simulink model "sim_stateEstimator"  (R2023b)
settings: Solver=VariableStepAuto  StartTime=0.0  StopTime=TSim  RelTol=1e-3
undefined symbols (not defined in the file): A, B, C, dampingCoeff, freqDist, initPos, initVel, K, l, magDist, mass, phaseDist, springCoeff
libraries: simulink x2
settings Model: Creator=uos  LastModifiedBy=hblee

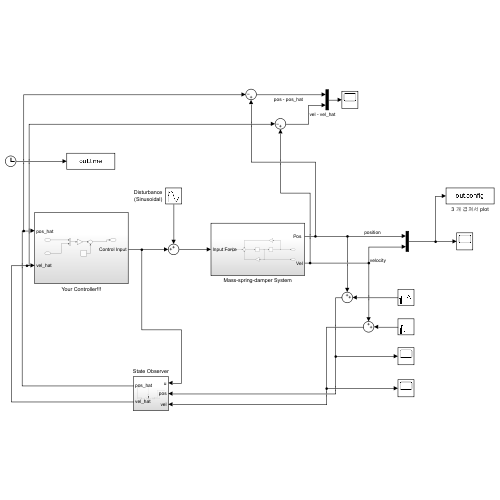
[thumbnail: Simulink's stored preview of the top-level diagram]
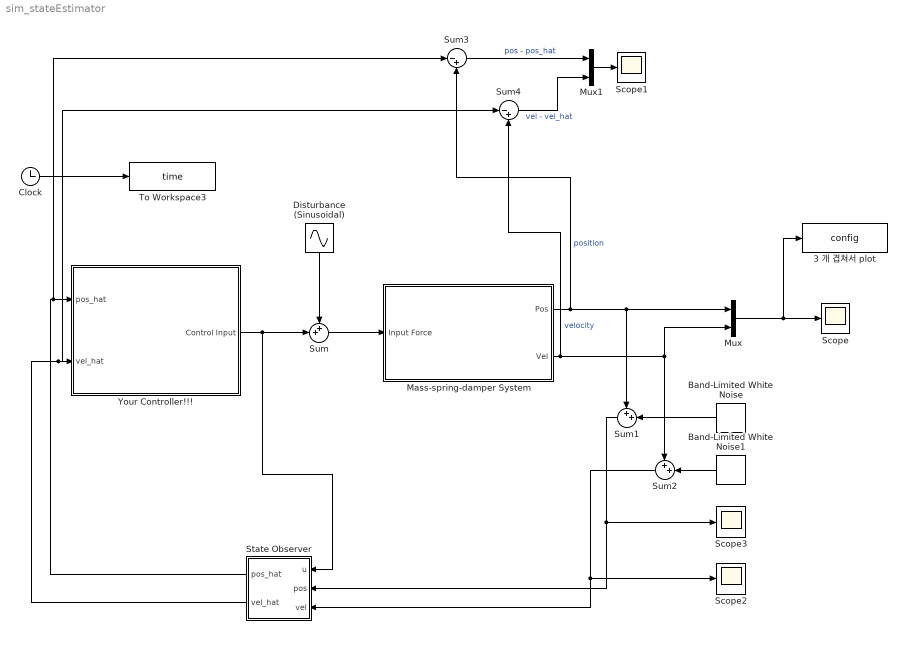
== system sim_stateEstimator ==
  3 개 겹쳐서 plot : ToWorkspace  VariableName=config  SampleTime=-1
  Band-Limited White Noise : simulink/Sources/Band-Limited White Noise  Cov=powerNoise  Ts=0.001  seed=[23341]
  Band-Limited White Noise1 : simulink/Sources/Band-Limited White Noise  Cov=powerNoise  Ts=0.001  seed=[23341]
  Clock : Clock
  Disturbance (Sinusoidal) : Sin  Amplitude=magDist  Bias=phaseDist  Frequency=freqDist  SampleTime=0
  Mass-spring-damper System : Subsystem
  Mux : Mux  Inputs=2
  Mux1 : Mux  Inputs=2
  Scope{,1..3} (4 alike) : Scope
  State Observer : Subsystem
  Sum : Sum  Inputs=++|
  Sum1 : Sum  Inputs=++|
  Sum2 : Sum  Inputs=++|
  Sum3 : Sum  Inputs=|-+
  Sum4 : Sum  Inputs=|-+
  To Workspace3 : ToWorkspace  VariableName=time  SampleTime=-1
  Your Controller!!! : Subsystem
  wires:
  Mass-spring-damper System/2(Vel) -> Mux/2, Sum2/1, Sum4/2  "velocity"
  Sum/1 -> Mass-spring-damper System/1("Input Force ")
  Your Controller!!!/1(Control Input) -> Sum/2, State Observer/1(u)
  Sum1/1 -> State Observer/2(pos), Scope3/1
  Sum2/1 -> State Observer/3(vel), Scope2/1
  Band-Limited White Noise/1 -> Sum1/2
  Band-Limited White Noise1/1 -> Sum2/2
  Disturbance (Sinusoidal)/1 -> Sum/1
  Clock/1 -> To Workspace3/1
  Mass-spring-damper System/1("Pos ") -> Sum3/2, Sum1/1, Mux/1  "position"
  Mux/1 -> 3 개 겹쳐서 plot/1, Scope/1
  State Observer/1(pos_hat) -> Sum3/1, Your Controller!!!/1(pos_hat)
  State Observer/2(vel_hat) -> Sum4/1, Your Controller!!!/2(vel_hat)
  Mux1/1 -> Scope1/1
  Sum3/1 -> Mux1/1  "pos - pos_hat"
  Sum4/1 -> Mux1/2  "vel - vel_hat"

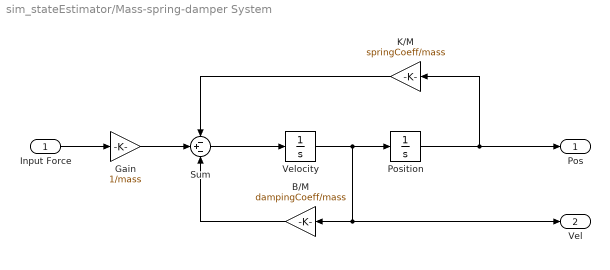
== system sim_stateEstimator/Mass-spring-damper System ==
  "Input Force " : Inport
  B/M : Gain  Gain=dampingCoeff/mass
  Gain : Gain  Gain=1/mass
  K/M : Gain  Gain=springCoeff/mass
  Position : Integrator  InitialCondition=initPos
  Sum : Sum  Inputs=-+-
  Velocity : Integrator  InitialCondition=initVel
  "Pos " : Outport
  Vel : Outport  Port=2
  wires:
  Velocity/1 -> Vel/1, B/M/1, Position/1
  Gain/1 -> Sum/2
  "Input Force "/1 -> Gain/1
  Position/1 -> "Pos "/1, K/M/1
  K/M/1 -> Sum/1
  B/M/1 -> Sum/3
  Sum/1 -> Velocity/1

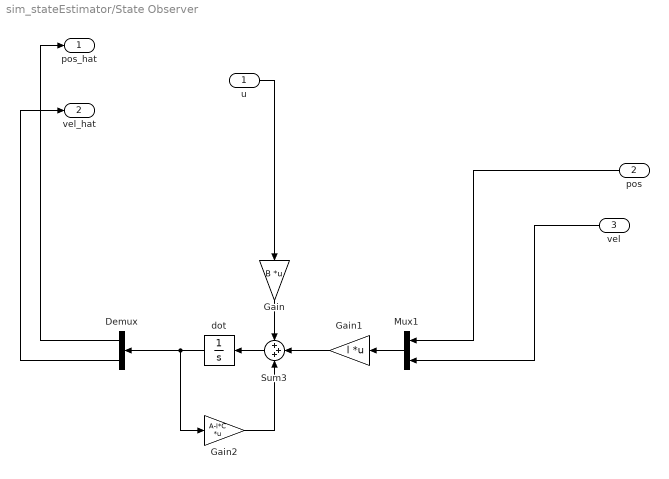
== system sim_stateEstimator/State Observer ==
  u : Inport
  pos : Inport  Port=2
  vel : Inport  Port=3
  Demux : Demux  Outputs=2
  Gain : Gain  Gain=B  Multiplication=Matrix(K*u)
  Gain1 : Gain  Gain=l  Multiplication=Matrix(K*u)
  Gain2 : Gain  Gain=A-l*C  Multiplication=Matrix(K*u)
  Mux1 : Mux  Inputs=2
  Sum3 : Sum  Inputs=+++
  dot : Integrator
  pos_hat : Outport
  vel_hat : Outport  Port=2
  wires:
  dot/1 -> Demux/1, Gain2/1
  pos/1 -> Mux1/1
  Mux1/1 -> Gain1/1
  Sum3/1 -> dot/1
  Gain2/1 -> Sum3/3
  Gain1/1 -> Sum3/2
  Gain/1 -> Sum3/1
  vel/1 -> Mux1/2
  Demux/2 -> vel_hat/1
  Demux/1 -> pos_hat/1
  u/1 -> Gain/1

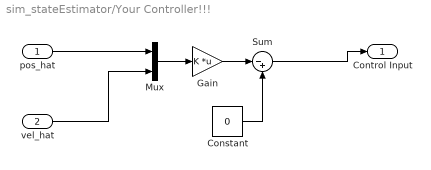
== system sim_stateEstimator/Your Controller!!! ==
  pos_hat : Inport
  vel_hat : Inport  Port=2
  Constant : Constant  Value=0
  Gain : Gain  Gain=K  Multiplication=Matrix(K*u)
  Mux : Mux  Inputs=2
  Sum : Sum  Inputs=|-+
  Control Input : Outport
  wires:
  Mux/1 -> Gain/1
  Gain/1 -> Sum/1
  Sum/1 -> Control Input/1
  Constant/1 -> Sum/2
  pos_hat/1 -> Mux/1
  vel_hat/1 -> Mux/2
